simulink model "m20p4"  (R2021b)
settings: Solver=ode45  StartTime=1  StopTime=100  FixedStep=0.1  RelTol=1e-3
undefined symbols (not defined in the file): nmax, nmax2, nmin, nmin2, seed, seed2, tc
settings Model: Creator=tanzc  LastModifiedBy=tanzc
settings DataIOCC: SaveFormat=Array  ReturnWorkspaceOutputs=off

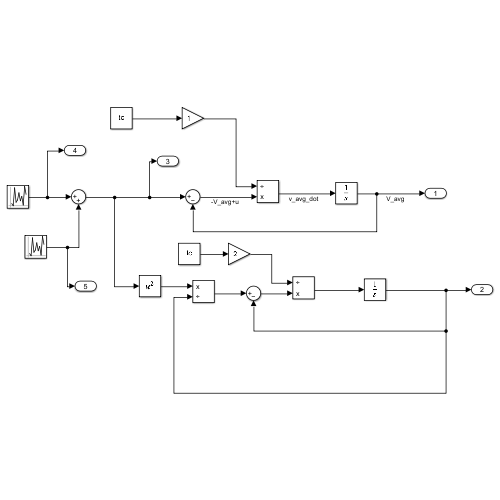
[thumbnail: Simulink's stored preview of the top-level diagram]
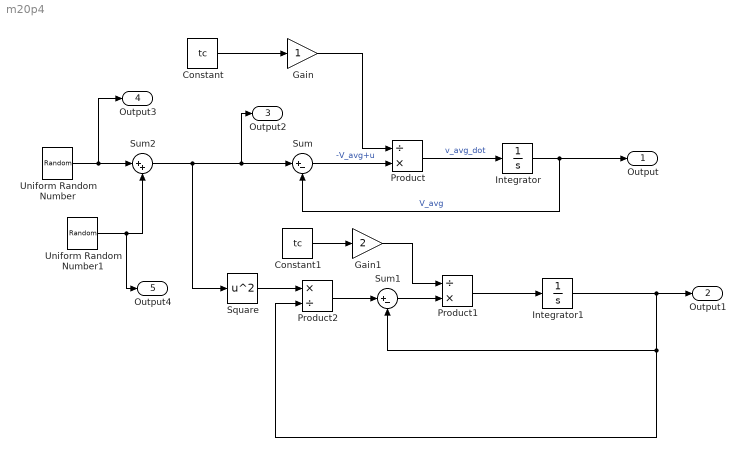
== system m20p4 ==
  Constant : Constant  Value=tc
  Constant1 : Constant  Value=tc
  Gain : Gain
  Gain1 : Gain  Gain=2
  Integrator : Integrator  InitialCondition=0.0001
  Integrator1 : Integrator  InitialCondition=0.0001
  Product : Product  Inputs=/*
  Product1 : Product  Inputs=/*
  Product2 : Product  Inputs=*/
  Square : Math  Operator=square  SaturateOnIntegerOverflow=on
  Sum : Sum  Inputs=|+-
  Sum1 : Sum  Inputs=|+-
  Sum2 : Sum  Inputs=|++
  Uniform Random Number : UniformRandomNumber  Minimum=nmin  Maximum=nmax  Seed=seed  SampleTime=1
  Uniform Random Number1 : UniformRandomNumber  Minimum=nmin2  Maximum=nmax2  Seed=seed2  SampleTime=1
  Output : Outport
  Output1 : Outport  Port=2
  Output2 : Outport  Port=3
  Output3 : Outport  Port=4
  Output4 : Outport  Port=5
  wires:
  Integrator/1 -> Output/1, Sum/2  "V_avg"
  Product/1 -> Integrator/1  "v_avg_dot"
  Constant/1 -> Gain/1
  Gain/1 -> Product/1
  Sum/1 -> Product/2  "-V_avg+u"
  Product1/1 -> Integrator1/1
  Constant1/1 -> Gain1/1
  Gain1/1 -> Product1/1
  Square/1 -> Product2/1
  Product2/1 -> Sum1/1
  Integrator1/1 -> Output1/1, Product2/2, Sum1/2
  Sum1/1 -> Product1/2
  Uniform Random Number1/1 -> Output4/1, Sum2/2
  Uniform Random Number/1 -> Output3/1, Sum2/1
  Sum2/1 -> Square/1, Output2/1, Sum/1
